simulink model "singen"  (Simulink 7.6)
settings: Solver=FixedStepDiscrete  SolverMode=SingleTasking  StartTime=0.0  StopTime=4e-6  RelTol=1e-3
InitFcn:
  | %% DSPBuilder Start
  | alt_dspbuilder_update_model(bdroot)
  | %% DSPBuilder End
libraries: allblocks_alteradspbuilder2 x13
settings Model: Creator=akarapet  LastModifiedBy=akarapet
settings DataIOCC: SignalLoggingName=sigsOut
settings OptimizationCC: BlockReduction=off  BooleanDataType=off  InlineInvariantSignals=on  InitFltsAndDblsToZero=on
settings DebuggingCC: SaveWithParameterizedLinksMsg=none  SignalResolutionControl=TryResolveAllWithWarning  SolverPrmCheckMsg=none  MultiTaskDSMMsg=warning  MultiTaskCondExecSysMsg=none  StrictBusMsg=None
settings HardwareCC: TargetUnknown=on
settings RTWCC: IncludeERTFirstTime=on
settings GRTTargetCC: TargetFcnLib=ansi_tfl_tmw.mat

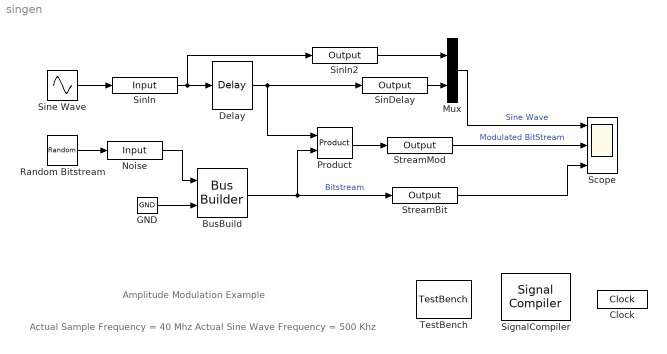
== system singen ==
  note: Amplitude Modulation Example
  note: Actual Sample Frequency = 40 Mhz
      | Actual Sine Wave Frequency = 500 Khz
  BusBuild : allblocks_alteradspbuilder2/Bus Builder  BusType=Signed Integer  bwl=2  bwr=0  pipeline_display=0
  Clock : allblocks_alteradspbuilder2/Clock  ClockPeriod=25  ClockPeriodUnit=ns  SampleTime=2.5e-008  ResetLatency=0  ResetRegisterCascadeDepth=0  SimulationStartCycle=5  PhaseOffset=0  Reset=aclr  ResetType=Active Low  Export=off
  Delay : allblocks_alteradspbuilder2/Delay  pipeline=1  pipeline_display=1  ClockPhase=01  use_ena=off  use_sclr=off  allowFloatingPointOverride=on  logOutputs=off  logFile=/data/akarapet/qshell_linux64_test/p4/dsp_builder/dsp_builder2/Documentation/DesignExamples/Tutorials/GettingStartedSinMdl/tb_singen/singen_Delay.fixedpointlog  use_init=off  reset_value=1
  GND : allblocks_alteradspbuilder2/GND  SpecifyClock=off
  Mux : Mux  Inputs=2
  Noise : allblocks_alteradspbuilder2/Input  iofile=/data/akarapet/qshell_linux64_test/p4/dsp_builder/dsp_builder2/Documentation/DesignExamples/Tutorials/GettingStartedSinMdl/tb_singen/singen_Noise.salt  BusType=Single Bit  bwl=1  bwr=0  SpecifyClock=off  PORTTYPE=Input  externalType=Inferred  allowFloatingPointOverride=on  logOutputs=off
  Product : allblocks_alteradspbuilder2/Product  BusType=Inferred  bwl=8  bwr=0  pipeline=0  pipeline_display=0  phase_selection=1  use_ena=off  use_aclr=off  UseLPM=off  UseDedicatedCircuitry=off  allowFloatingPointOverride=on  logOutputs=off  logFile=/data/akarapet/qshell_linux64_test/p4/dsp_builder/dsp_builder2/Documentation/DesignExamples/Tutorials/GettingStartedSinMdl/tb_singen/singen_Product.fixedpointlog
  Random Bitstream : RandomNumber  SampleTime=25e-9
  Scope : Scope  NumInputPorts=3
      settings: TimeRange=23.41356673960612  YMin=-5512.82~-5~-5  YMax=8076.92~5~5
  SignalCompiler : allblocks_alteradspbuilder2/Signal Compiler  DeviceFamily=Stratix III  DeviceName=AUTO  EnableSignalTap=off  SignalTapDepth=128  UseBoardBlock=off  StpUseDefaultClock=on  StpClock=Clock  ExportDir=<binary blob, 122 chars, not shown>
  SinDelay : allblocks_alteradspbuilder2/Output  iofile=/data/akarapet/qshell_linux64_test/p4/dsp_builder/dsp_builder2/Documentation/DesignExamples/Tutorials/GettingStartedSinMdl/tb_singen/singen_SinDelay.capture  BusType=Signed Integer  bwl=16  bwr=0  externalType=Inferred  PORTTYPE=Output  allowFloatingPointOverride=on  logOutputs=off
  SinIn : allblocks_alteradspbuilder2/Input  iofile=/data/akarapet/qshell_linux64_test/p4/dsp_builder/dsp_builder2/Documentation/DesignExamples/Tutorials/GettingStartedSinMdl/tb_singen/singen_SinIn.salt  BusType=Signed Integer  bwl=16  bwr=0  SpecifyClock=off  PORTTYPE=Input  externalType=Inferred  allowFloatingPointOverride=on  logOutputs=off
  SinIn2 : allblocks_alteradspbuilder2/Output  iofile=/data/akarapet/qshell_linux64_test/p4/dsp_builder/dsp_builder2/Documentation/DesignExamples/Tutorials/GettingStartedSinMdl/tb_singen/singen_SinIn2.capture  BusType=Signed Integer  bwl=16  bwr=0  externalType=Inferred  PORTTYPE=Output  allowFloatingPointOverride=on  logOutputs=off
  Sine Wave : Sin  SineType=Sample based  Amplitude=2^15-1  Frequency=500e3*2*pi  Samples=80  SampleTime=25e-9
  StreamBit : allblocks_alteradspbuilder2/Output  iofile=/data/akarapet/qshell_linux64_test/p4/dsp_builder/dsp_builder2/Documentation/DesignExamples/Tutorials/GettingStartedSinMdl/tb_singen/singen_StreamBit.capture  BusType=Single Bit  bwl=19  bwr=0  externalType=Inferred  PORTTYPE=Output  allowFloatingPointOverride=on  logOutputs=off
  StreamMod : allblocks_alteradspbuilder2/Output  iofile=/data/akarapet/qshell_linux64_test/p4/dsp_builder/dsp_builder2/Documentation/DesignExamples/Tutorials/GettingStartedSinMdl/tb_singen/singen_StreamMod.capture  BusType=Signed Integer  bwl=19  bwr=0  externalType=Inferred  PORTTYPE=Output  allowFloatingPointOverride=on  logOutputs=off
  TestBench : allblocks_alteradspbuilder2/TestBench  enable=on  advancedMode=off  modelSimGui=off  maxDisplayErrors=10  mismatchErrorLevel=Error  simdatafile=/data/akarapet/qshell_linux64_test/p4/dsp_builder/dsp_builder2/Documentation/DesignExamples/Tutorials/GettingStartedSinMdl/tb_singen/singen.simdata.tcl
  wires:
  Sine Wave/1 -> SinIn/1
  SinIn/1 -> Delay/1, SinIn2/1
  Delay/1 -> Product/1, SinDelay/1
  SinDelay/1 -> Mux/2
  Random Bitstream/1 -> Noise/1
  Product/1 -> StreamMod/1
  Noise/1 -> BusBuild/1
  BusBuild/1 -> Product/2, StreamBit/1  "Bitstream"
  StreamMod/1 -> Scope/2  "Modulated BitStream"
  Mux/1 -> Scope/1  "Sine Wave"
  GND/1 -> BusBuild/2
  StreamBit/1 -> Scope/3
  SinIn2/1 -> Mux/1
